simulink model "am"  (R2020b)
settings: Solver=VariableStepAuto  StartTime=0.0  StopTime=0.01  RelTol=1e-3
libraries: dspsrcs4 x2, dsparch4 x1
settings Model: Creator=tamim  LastModifiedBy=tamim
settings DebuggingCC: SFMachineParentedDataDiag=error

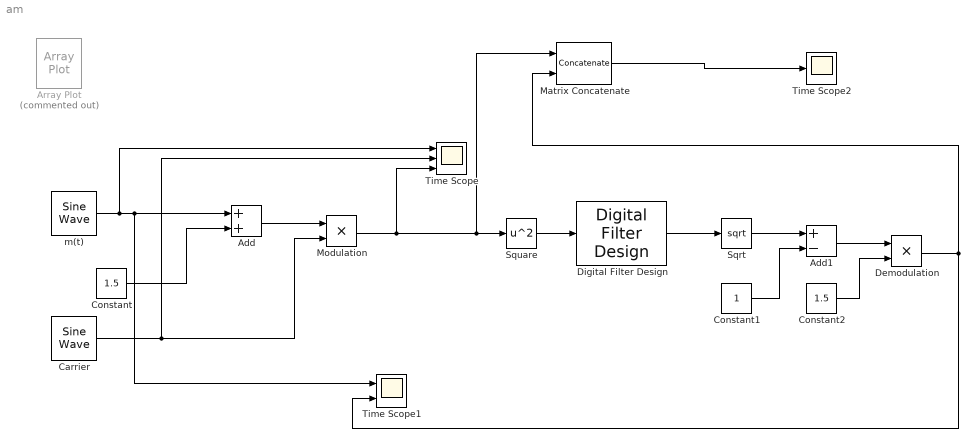
== system am ==
  Add : Sum
  Add1 : Sum  Inputs=+-
  Array Plot : ArrayPlot  Commented=on  DefaultConfigurationName=dsp.scopes.ArrayPlotBlockSpecification
  Carrier : dspsrcs4/Sine Wave  Amplitude=1  Frequency=15000  Phase=0  SampleMode=Discrete  OutComplex=Real  CompMethod=Trigonometric fcn  TableSize=Speed  SampleTime=1/96000  SamplesPerFrame=64  ResetState=Restart at time zero  OutputFrames=off  dataType=double  wordLen=16  udDataType=sfix(16)  fracBitsMode=Best precision  numFracBits=15  OutDataTypeStr=double  LastOutDataTypeStr=double
  Constant : Constant  Value=1.5
  Constant1 : Constant
  Constant2 : Constant  Value=1.5
  Demodulation : Product
  Digital Filter Design : dsparch4/Digital Filter Design  mwdsp_browser_bugfix_var=off
  Matrix Concatenate : Concatenate  Mode=Multidimensional array  ConcatenateDimension=2
  Modulation : Product
  Sqrt : Sqrt  SaturateOnIntegerOverflow=on
  Square : Math  Operator=square  SaturateOnIntegerOverflow=on
  Time Scope : Scope  NumInputPorts=3
  Time Scope1 : Scope  NumInputPorts=2
  Time Scope2 : Scope
  m(t) : dspsrcs4/Sine Wave  Amplitude=1  Frequency=1000  Phase=0  SampleMode=Discrete  OutComplex=Real  CompMethod=Trigonometric fcn  TableSize=Speed  SampleTime=1/96000  SamplesPerFrame=64  ResetState=Restart at time zero  OutputFrames=off  dataType=double  wordLen=16  udDataType=sfix(16)  fracBitsMode=Best precision  numFracBits=15  OutDataTypeStr=double  LastOutDataTypeStr=double
  wires:
  m(t)/1 -> Time Scope1/1, Add/1, Time Scope/1
  Constant/1 -> Add/2
  Add/1 -> Modulation/1
  Carrier/1 -> Time Scope/2, Modulation/2
  Modulation/1 -> Matrix Concatenate/1, Square/1, Time Scope/3
  Square/1 -> Digital Filter Design/1
  Digital Filter Design/1 -> Sqrt/1
  Sqrt/1 -> Add1/1
  Constant1/1 -> Add1/2
  Add1/1 -> Demodulation/1
  Constant2/1 -> Demodulation/2
  Demodulation/1 -> Matrix Concatenate/2, Time Scope1/2
  Matrix Concatenate/1 -> Time Scope2/1
